simulink model "dir_lmap"  (R2018b)
settings: Solver=FixedStepDiscrete  StartTime=0.0  StopTime=10.0  FixedStep=0.01  RelTol=1e-3
settings Model: Creator=roberto  LastModifiedBy=roberto
settings OptimizationCC: DefaultParameterBehavior=Inlined  EnhancedBackFolding=on  PassReuseOutputArgsAs=Individual arguments  OptimizeBlockOrder=speed  DifferentSizesBufferReuse=on  OptimizationCustomize=off
settings DebuggingCC: ParameterTunabilityLossMsg=error
settings SFSimCC: MATLABDynamicMemAlloc=off
settings RTWCC: SystemTargetFile=ert.tlc  GenCodeOnly=on  TemplateMakefile=ert_default_tmf  GenerateReport=on  IncludeHyperlinkInReport=on  LaunchReport=on  GenerateTraceInfo=on  GenerateTraceReport=on  GenerateTraceReportSl=on  GenerateTraceReportSf=on  GenerateTraceReportEml=on  GenerateCodeMetricsReport=on
settings CodeAppCC: ForceParamTrailComments=on  IgnoreCustomStorageClasses=off  OperatorAnnotations=on  SimulinkDataObjDesc=on  SFDataObjDesc=on  InsertBlockDesc=on
settings ERTTargetCC: TargetLangStandard=C99 (ISO)  GenerateSampleERTMain=on  InlinedParameterPlacement=NonHierarchical  ERTCustomFileTemplate=example_file_process.tlc

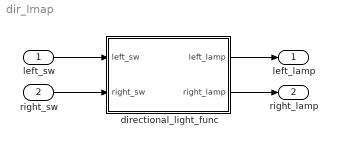
== system dir_lmap ==
  left_sw : Inport  OutDataTypeStr=boolean
  right_sw : Inport  Port=2  OutDataTypeStr=boolean
  directional_light_func : Subsystem  TreatAsAtomicUnit=on
      settings: RTWFcnNameOpts=Use subsystem name  RTWFileNameOpts=Use subsystem name
  left_lamp : Outport  OutDataTypeStr=boolean
  right_lamp : Outport  Port=2  OutDataTypeStr=boolean
  wires:
  left_sw/1 -> directional_light_func/1(left_sw)
  directional_light_func/1(left_lamp) -> left_lamp/1
  directional_light_func/2(right_lamp) -> right_lamp/1
  right_sw/1 -> directional_light_func/2(right_sw)

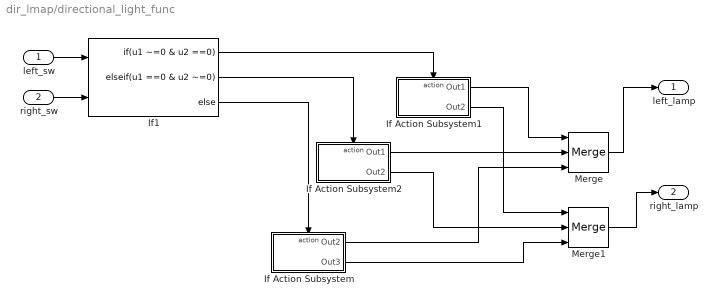
== system dir_lmap/directional_light_func ==
  left_sw : Inport  OutDataTypeStr=boolean
  right_sw : Inport  Port=2  OutDataTypeStr=boolean
  If Action Subsystem : Subsystem  TreatAsAtomicUnit=on
  If Action Subsystem1 : Subsystem  TreatAsAtomicUnit=on
  If Action Subsystem2 : Subsystem  TreatAsAtomicUnit=on
  If1 : If  NumInputs=2  IfExpression=u1 ~=0 & u2 ==0  ElseIfExpressions=u1 ==0 & u2 ~=0
  Merge : Merge  Inputs=3
  Merge1 : Merge  Inputs=3
  left_lamp : Outport  OutDataTypeStr=boolean
  right_lamp : Outport  Port=2  OutDataTypeStr=boolean
  wires:
  left_sw/1 -> If1/1
  right_sw/1 -> If1/2
  If1/1 -> If Action Subsystem1/Action
  If1/2 -> If Action Subsystem2/Action
  If1/3 -> If Action Subsystem/Action
  If Action Subsystem1/1(Out1) -> Merge/1
  If Action Subsystem2/1(Out1) -> Merge/2
  If Action Subsystem/1(Out2) -> Merge/3
  Merge/1 -> left_lamp/1
  If Action Subsystem1/2(Out2) -> Merge1/1
  If Action Subsystem2/2(Out2) -> Merge1/2
  If Action Subsystem/2(Out3) -> Merge1/3
  Merge1/1 -> right_lamp/1

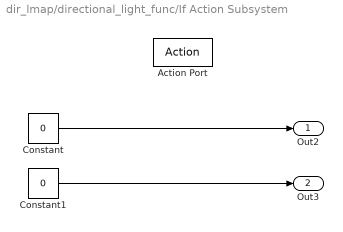
== system dir_lmap/directional_light_func/If Action Subsystem ==
  Action Port : ActionPort  ActionType=else
  Constant : Constant  Value=0  OutDataTypeStr=boolean
  Constant1 : Constant  Value=0  OutDataTypeStr=boolean
  Out2 : Outport
  Out3 : Outport  Port=2
  wires:
  Constant/1 -> Out2/1
  Constant1/1 -> Out3/1

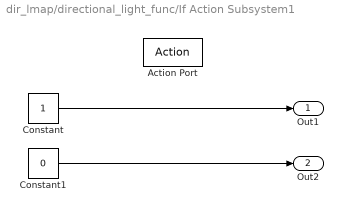
== system dir_lmap/directional_light_func/If Action Subsystem1 ==
  Action Port : ActionPort  ActionType=then
  Constant : Constant  OutDataTypeStr=boolean
  Constant1 : Constant  Value=0  OutDataTypeStr=boolean
  Out1 : Outport
  Out2 : Outport  Port=2
  wires:
  Constant/1 -> Out1/1
  Constant1/1 -> Out2/1

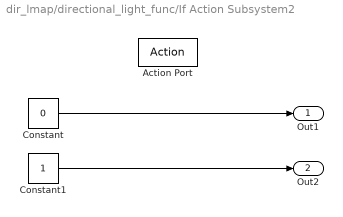
== system dir_lmap/directional_light_func/If Action Subsystem2 ==
  Action Port : ActionPort  ActionType=elseif
  Constant : Constant  Value=0  OutDataTypeStr=boolean
  Constant1 : Constant  OutDataTypeStr=boolean
  Out1 : Outport
  Out2 : Outport  Port=2
  wires:
  Constant/1 -> Out1/1
  Constant1/1 -> Out2/1
